simulink model "PLFrameGenerator"  (R2023a)
settings: Solver=FixedStepAuto  StartTime=0.0  StopTime=135e-7  RelTol=1e-3
model workspace (MAT data in the model file):
  G = [1  0  0  1  0  0  0  0  1  0  1  0  1  1  0  0  0  0  1  0  1  1  0  1  1  1  0  1  1  1  0  1; 0  1  0  1  0  1  0  1  0  1  0  1  0  1  0  1  0  1  0  1  0  1  0  1  0  1  0  1  0  1  0  1; 0  0  1  1  0  0  1  1  0  0  1  1  0  0  1  1  0  0  1  1  0  0  1  1  0  0  1  1  0  0  1  1; 0  0  0  0  1  1  1  1  0  0  0  0  1  1  1  1  0  0  0  0  1  1  1  1  0  0  0  0  1  1  1  1; 0  0  0  0  0  0  0  0  1  1  1  1  1  1  1  1  0  0  0  0  0  0  0  0  1  1  1  1  1  1  1  1; 0  0  0  0  0  0  0  0  0  0  0  0  0  0  0  0  1  1  1  1  1  1  1  1  1  1  1  1  1  1  1  1; 1  1  1  1  1  1  1  1  1  1  1  1  1  1  1  1  1  1  1  1  1  1  1  1  1  1  1  1  1  1  1  1]
  HDRShortDUMMY = Simulink.LookupTable
  HDRShortDUMMY.Table = Simulink.lookuptable.Table
  HDRShortDUMMY.Table.Value = [-0.707106781187-0.707106781187i -0.707106781187+0.707106781187i -0.707106781187-0.707106781187i 0.707106781187-0.707106781187i -0.707106781187-0.707106781187i 0.707106781187-0.707106781187i 0.707106781187+0.707106781187i -0.707106781187+0.707106781187i 0.707106781187+0.707106781187i -0.707106781187+0.707106781187i 0.707106781187+0.707106781187i 0.707106781187-0.707106781187i ... (64 elements, 64x1)]
  HDRShortDUMMY.Table.Dimensions = [64 1]
  HDRShortDUMMY.Table.DataType = 'auto'
  HDRShortDUMMY.Table.FieldName = 'Table'
  HDRShortDUMMY.Breakpoints = Simulink.lookuptable.Breakpoint
  HDRShortDUMMY.Breakpoints.TunableSizeName = 'N1'
  HDRShortDUMMY.Breakpoints.Dimensions = [0 0]
  HDRShortDUMMY.Breakpoints.DataType = 'auto'
  HDRShortDUMMY.Breakpoints.FieldName = 'BP1'
  HDRShortDUMMY.AllowMultipleInstancesOfTypeToHaveDifferentTableBreakpointSizes = 0
  HDRShortDUMMY.SupportTunableSize = 0
  HDRShortDUMMY.StructTypeInfo = Simulink.lookuptable.StructTypeInfo
  HDRShortDUMMY.StructTypeInfo.DataScope = 'Auto'
  PLSCLength = 90
  PilotMaxIdx = 1475
  PilotMinIdx = 1440
  Rsym = 10000000
  SNR = Simulink.Parameter
  SNR.Value = 50
  SNR.DataType = 'auto'
  SNR.Complexity = 'real'
  SNR.Dimensions = [1 1]
  SOFLength = 26
  debugHeaderGain = 2
  mwTaskManagerKernelLatency = 0
  up_coef = 2
undefined symbols (not defined in the file or in its folder): Add, magnitude, Shift
libraries: simulink x15, hdlsllib x14, dsphdlfiltering2 x4, embmathops x4, dspsigops x3, commrandsrc3 x1, commfilt2 x1, dsphdlmathfun2 x1, commchan3 x1
(part 1 of 2)
settings Model: SimulationMode=accelerator  ParameterArgumentNames=SNR  Creator=svdvl  LastModifiedBy=x
settings OptimizationCC: DefaultParameterBehavior=Inlined  EnhancedBackFolding=on  PassReuseOutputArgsAs=Individual arguments  ZeroExternalMemoryAtStartup=off  ZeroInternalMemoryAtStartup=off  MaxStackSize=64  OptimizeBlockOrder=speed  DifferentSizesBufferReuse=on  OptimizationCustomize=off  EfficientTunableParamExpr=on
settings DebuggingCC: SingleTaskRateTransMsg=error  ParameterTunabilityLossMsg=error
settings HardwareCC: ProdBitPerPointer=32  ProdBitPerSizeT=32  ProdBitPerPtrDiffT=32  ProdLargestAtomicFloat=None  ProdIntDivRoundTo=Undefined  ProdEndianess=Unspecified  ProdWordSize=32  ProdHWDeviceType=ASIC/FPGA->ASIC/FPGA  TargetBitPerPointer=64  TargetBitPerSizeT=64  TargetBitPerPtrDiffT=64  TargetLongLongMode=on  TargetIntDivRoundTo=Zero  TargetEndianess=LittleEndian  TargetWordSize=64  TargetHWDeviceType=Custom Processor->MATLAB Host Computer  ProdEqTarget=off  HardwareBoardFeatureSet=SoCBlockset
settings SFSimCC: MATLABDynamicMemAlloc=off
settings RTWCC: Description=Embedded Coder  SystemTargetFile=ert.tlc  HardwareBoard=Xilinx Kintex-7 KC705 development board  TemplateMakefile=ert_default_tmf
settings CodeAppCC: ForceParamTrailComments=on  IgnoreCustomStorageClasses=off  OperatorAnnotations=on  SimulinkDataObjDesc=on  SFDataObjDesc=on  InsertBlockDesc=on
settings ERTTargetCC: InlinedParameterPlacement=NonHierarchical

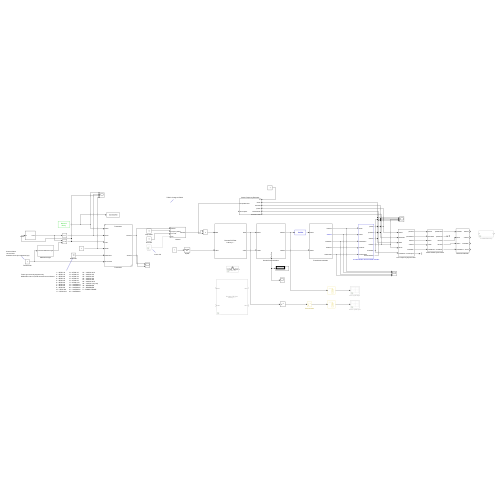
[thumbnail: Simulink's stored preview of the top-level diagram]
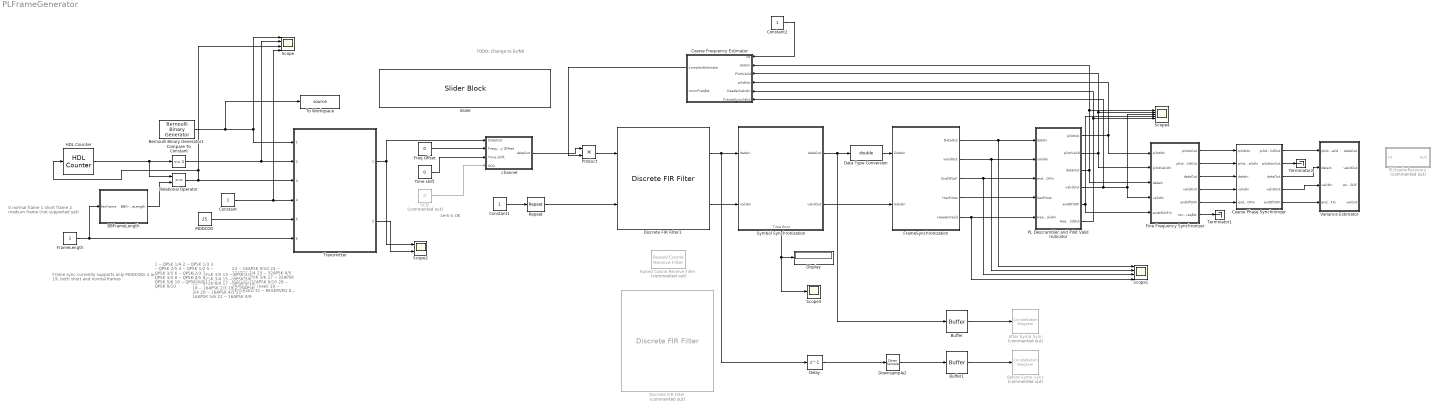
== system PLFrameGenerator ==
  note: Frame sync currently supports only
      | MODCODs 4 and 19, both short and normal frames
  note: 1e-6 is OK
  note: TODO: Change to Es/N0
  note: 23 -- 16APSK 9/10
      | 24 -- 32APSK 3/4
      | 25 -- 32APSK 4/5
      | 26 -- 32APSK 5/6
      | 27 -- 32APSK 8/9
      | 28 -- 32APSK 9/10
      | 29 -- 16APSK 1/2 (new)
      | 30 -- RESERVED
      | 31 -- RESERVED
      | 0 -- DUMMY FRAME
  note: 12 -- 8PSK 3/5
      | 13 -- 8PSK 2/3
      | 14 -- 8PSK 3/4
      | 15 -- 8PSK 5/6
      | 16 -- 8PSK 8/9
      | 17 -- 8PSK 9/10
      | 18 -- 16APSK 2/3
      | 19 -- 16APSK 3/4
      | 20 -- 16APSK 4/5
      | 21 -- 16APSK 5/6
      | 22 -- 16APSK 8/9
  note: 1 -- QPSK 1/4
      | 2 -- QPSK 1/3
      | 3 -- QPSK 2/5
      | 4 -- QPSK 1/2
      | 5 -- QPSK 3/5
      | 6 -- QPSK 2/3
      | 7 -- QPSK 3/4
      | 8 -- QPSK 4/5
      | 9 -- QPSK 5/6
      | 10 -- QPSK 8/9
      | 11 -- QPSK 9/10
  note: 0 normal frame
      | 1 short frame
      | 2 medium frame (not supported yet)
  After Symb Sync : ConstellationDiagram  Commented=on  WindowPosition=[1126.000000,74.000000,600.000000,600.000000,]  ScopeFrameLocation=window  DefaultConfigurationName=comm.scopes.ConstellationDiagramBlockCfg
  BBFrameLength : Subsystem
  Before Symb Sync : ConstellationDiagram  Commented=on  WindowPosition=[70.000000,95.000000,600.000000,600.000000,]  ScopeFrameLocation=window  DefaultConfigurationName=comm.scopes.ConstellationDiagramBlockCfg
  Bernoulli Binary Generator1 : commrandsrc3/Bernoulli Binary Generator  ProbabilityOfZero=0.5  SeedSource=Auto  Seed=0  SampleTime=1/Rsym/8  SamplesPerFrame=1  OutputDataType=boolean  SimulateUsing=Code generation
  Buffer : Buffer  N=1000  OutputFrames=off
  Buffer1 : Buffer  N=1000  OutputFrames=off
  Coarse Frequency Estimator : Subsystem
  Coarse Phase Synchronizer : Subsystem
  Compare To Constant : simulink/Logic and Bit Operations/Compare To Constant  relop===  const=1  OutDataTypeStr=boolean
  Constant : Constant  OutDataTypeStr=boolean  SampleTime=1/Rsym/8
  Constant1 : Constant  OutDataTypeStr=boolean  SampleTime=-1
  Constant2 : Constant  SampleTime=-1
  Data Type Conversion : DataTypeConversion  OutDataTypeStr=double  SaturateOnIntegerOverflow=off  RndMeth=Floor
  Delay : Delay  DelayLength=1
  Discrete FIR Filter : dsphdlfiltering2/Discrete FIR Filter  Commented=on  NumeratorSource=Property  Numerator="[-0.00285820997079789\t0.00137733032508190\t0.00315455482520775\t-0.00356415296709377\t-0.00206211933009069\t0.00514477794743620\t-0.000825518525453186\t-0.00481272795526686\t0.00560922270003514\t0.000910808542107733\t-0.0120044818773511\t0.00862996822246556\t0.0193455321229390\t-0.0268242332250627\t-0.0266806119948057\t0.0600224093867556\t0.0329422984385442\t-0.130628932045810\t-0.0371565869289195\t0.443442194227448\t0.745765109300838\t0.443442194227448\t-0.0371565869289195\t-0.130628932045810\t0.0329422984385442\t0.0600224093867556\t-0.0266806119948057\t-0.0268242332250627\t0.0193455321229390\t0.00862996822246556\t-0.0120044818773511\t0.000910808542107733\t0.00560922270003514\t-0.00481272795526686\t-0.000825518525453186\t0.00514477794743620\t-0.00206211933009069\t-0.00356415296709377\t0.00315455482520775\t0.00137733032508190\t-0.00285820997079789]"  NumeratorPrototype=[]  FilterStructure=Direct form systolic  SerializationOption=Minimum number of cycles between valid input samples  NumCycles=2  NumberOfMultipliers=2  SimulateUsing=Code generation  roundingMode=Floor  overflowMode=off  CoefficientsDataTypeStr=Inherit: Same word length as input  OutputDataTypeStr=Inherit: Same word length as input  ResetInputPort=off  HDLGlobalReset=off
  Discrete FIR Filter1 : dsphdlfiltering2/Discrete FIR Filter  NumeratorSource=Property  Numerator="[-0.00285820997079789\t0.00137733032508190\t0.00315455482520775\t-0.00356415296709377\t-0.00206211933009069\t0.00514477794743620\t-0.000825518525453186\t-0.00481272795526686\t0.00560922270003514\t0.000910808542107733\t-0.0120044818773511\t0.00862996822246556\t0.0193455321229390\t-0.0268242332250627\t-0.0266806119948057\t0.0600224093867556\t0.0329422984385442\t-0.130628932045810\t-0.0371565869289195\t0.443442194227448\t0.745765109300838\t0.443442194227448\t-0.0371565869289195\t-0.130628932045810\t0.0329422984385442\t0.0600224093867556\t-0.0266806119948057\t-0.0268242332250627\t0.0193455321229390\t0.00862996822246556\t-0.0120044818773511\t0.000910808542107733\t0.00560922270003514\t-0.00481272795526686\t-0.000825518525453186\t0.00514477794743620\t-0.00206211933009069\t-0.00356415296709377\t0.00315455482520775\t0.00137733032508190\t-0.00285820997079789]"  NumeratorPrototype=[]  FilterStructure=Direct form systolic  SerializationOption=Minimum number of cycles between valid input samples  NumCycles=2  NumberOfMultipliers=2  SimulateUsing=Code generation  roundingMode=Floor  overflowMode=off  CoefficientsDataTypeStr=Inherit: Same word length as input  OutputDataTypeStr=Inherit: Same word length as input  ResetInputPort=off  HDLGlobalReset=off
  Display : Display
  Downsample2 : DownSample  RateOptions=Allow multirate processing
  Fine Frequency Synchronizer : Subsystem
  FrameLength : Constant  OutDataTypeStr=fixdt(0,2,0)  SampleTime=1/Rsym/8
  FrameSynchronization : Subsystem
  Freq Offset : Constant  Value=0
  HDL Counter : hdlsllib/Sources/HDL Counter  CountType=Count limited  CountInit=1  CountStep=1  CountMax=64800  CountFromType=Initial value  CountFrom=1  CountResetPort=on  CountLoadPort=off  CountEnbPort=off  CountDirPort=off  CountHitOutputPort=off  CountDataType=Unsigned  CountWordLen=16  CountFracLen=0  CountSampTime=1/Rsym/8
  MODCOD : Constant  Value=25  VectorParams1D=off  OutDataTypeStr=fixdt(0, 5, 0)  SampleTime=1/Rsym/8
  PL Descrambler and Pilot Valid Indicator : Subsystem
  PLHeaderRecovery : Subsystem  Commented=on
  Product : Product
  Raised Cosine Receive Filter : commfilt2/Raised Cosine Receive Filter  Commented=on  filtType=Square root  R=0.2  filtSpan=20  N=2  downFactor=1  downOffset=0  filterGain=1  InputProcessing=Columns as channels (frame based)  RateOptions=Enforce single-rate processing  framing=Mute  checkCoeff=on  variableName=rcRxFilt  currentFiltSpan=10  D=5  inputOffset=0  sampMode=Mute  saveAsFlag=0  rateMode=Downsampling  checkGain=Normalized  launchFVT=on  roundingMode=Floor  overflowMode=off  coeffDataTypeStr=Inherit: Same word length as input  coeffMin=[]  coeffMax=[]  coeffLastDataTypeStr=Inherit: Same word length as input  accumDataTypeStr=Inherit: Same as product output  accumLastDataTypeStr=Inherit: Same as product output  outputDataTypeStr=Inherit: Same as accumulator  outputMin=[]  outputMax=[]  outputLastDataTypeStr=Inherit: Same as accumulator
  Relational Operator : RelationalOperator  Operator===  OutDataTypeStr=boolean  RndMeth=Simplest  InputSameDT=off
  Repeat : dspsigops/Repeat  FactorSource=Dialog parameter  N=2  Nmax=16  RateOptions=Allow multirate processing  ic=0  mode=Unused parameter value
      settings: LibrarySourceBlock=dsphdlsupportsigops/Repeat
  SCO : Constant  Commented=on  Value=0  SampleTime=1/2/Rsym
  Scope : Scope  NumInputPorts=4
  Scope1 : Scope  NumInputPorts=4
  Scope2 : Scope  NumInputPorts=2
  Scope3 : Scope
  Scope4 : Scope  NumInputPorts=5
  Slider : SliderBlock  ScaleMin=-10  ScaleMax=50
  Symbol Synchronization : Subsystem
      settings: PortSchema="{\"entries\":[{\"content\":{\"sides\":[{\"content\":{\"connectorIds\":[\"In1\",\"In2\"]},\"type\":\"ConnectorPlacement.EquallySpacedRectSide\",\"uuid\":\"e58971f0-ac8c-4c81-a411-2548e0157a31\"},{\"content\":{\"connectorIds\":[\"Out1\",\"Out2\"],\"side\":\"RIGHT\"},\"type\":\"ConnectorPlacement.EquallySpacedRectSide\",\"uuid\":\"61e7e244-d935-4f43-ae64-0dd24601d7d6\"},{\"content\":{\"connectorIds\":[],\"side\":\"TOP\"},\"type\":\"ConnectorPlacement.EquallySpacedRectSide\",\"uuid\":\"96280ba8-4d2f-4f61-8153-d5e9f705abd5\"},{\"content\":{\"connectorIds\":[\"Out3\"],\"side\":\"BOTTOM\"},\"type\":\"ConnectorPlacement.EquallySpacedRectSide\",\"uuid\":\"1f39d276-a9ad-4a31-a5cc-29fbe76e4b28\"}]},\"type\":\"ConnectorPlacement.EquallySpacedConnector\",\"uuid\":\"475f41bb-1527-498a-b7fd-c47195976015\"}],\"packageUris\":[\"http://schema.mathworks.com/mf0/Connector/R2020b\"],\"version\":\"1.0\"}"
  Terminator1 : Terminator
  Terminator2 : Terminator
  Time shift : Constant  Value=0  SampleTime=-1
  To Workspace : ToWorkspace  VariableName=source  SampleTime=-1
  Transmitter : Subsystem  ReferencedSubsystem=Transmitter
  Variance Estimator : Subsystem
  channel : Subsystem
  wires:
  Bernoulli Binary Generator1/1 -> To Workspace/1, Transmitter/1, Scope/1
  Constant/1 -> Transmitter/4, Scope/4
  FrameLength/1 -> Transmitter/6, BBFrameLength/1(fecframe)
  Compare To Constant/1 -> Transmitter/2, Scope/2
  HDL Counter/1 -> Compare To Constant/1, Relational Operator/1
  BBFrameLength/1(BBFrameLength) -> Relational Operator/2
  MODCOD/1 -> Transmitter/5
  Relational Operator/1 -> Transmitter/3, Scope/3, HDL Counter/1
  Transmitter/1 -> Scope2/1, channel/1(DataOut)
  Transmitter/2 -> Scope2/2
  Constant1/1 -> Repeat/1
  Buffer/1 -> After Symb Sync/1
  Symbol Synchronization/1(dataOut) -> Data Type Conversion/1, Buffer/1
  FrameSynchronization/1(DataOut) -> Scope1/1, PL Descrambler and Pilot Valid Indicator/1(dataIn)
  FrameSynchronization/2(ValidOut) -> Scope1/2, PL Descrambler and Pilot Valid Indicator/2(validIn)
  FrameSynchronization/3(EndOfSoF) -> Scope1/3, PL Descrambler and Pilot Valid Indicator/3(endOfSOFIn)
  Data Type Conversion/1 -> FrameSynchronization/1(DataIn)
  Symbol Synchronization/2(validOut) -> FrameSynchronization/2(ValidIn)
  Freq Offset/1 -> channel/2(Frequency Offset)
  Time shift/1 -> channel/3(Time shift)
  SCO/1 -> channel/4(SCO)
  Buffer1/1 -> Before Symb Sync/1
  Downsample2/1 -> Buffer1/1
  Product/1 -> Discrete FIR Filter1/1
  Discrete FIR Filter1/1 -> Delay/1, Symbol Synchronization/1(dataIn)
  Discrete FIR Filter1/2 -> Symbol Synchronization/2(validIn)
  Repeat/1 -> Discrete FIR Filter1/2
  Delay/1 -> Downsample2/1
  Symbol Synchronization/3(Time Error) -> Scope3/1, Display/1
  FrameSynchronization/4(HasPilots) -> PL Descrambler and Pilot Valid Indicator/4(hasPilots)
  PL Descrambler and Pilot Valid Indicator/1(pilotIdx) -> Fine Frequency Synchronizer/1(pilotIdx), Coarse Frequency Estimator/4(pilotIdx)
  PL Descrambler and Pilot Valid Indicator/2(pilotValid) -> Fine Frequency Synchronizer/2(pilotValidIn), Coarse Frequency Estimator/3(PilotValid), Scope4/2
  PL Descrambler and Pilot Valid Indicator/3(dataOut) -> Coarse Frequency Estimator/2(dataIn), Scope4/1, Fine Frequency Synchronizer/3(dataIn)
  Constant2/1 -> Coarse Frequency Estimator/1(rst)
  Coarse Frequency Estimator/1(complexEstimate) -> Product/2
  PL Descrambler and Pilot Valid Indicator/4(validOut) -> Fine Frequency Synchronizer/4(validIn), Scope4/3, Coarse Frequency Estimator/6(FrameSyncValid)
  PL Descrambler and Pilot Valid Indicator/5(endOfSOF) -> Scope4/4, Fine Frequency Synchronizer/5(endofSOFIn)
  Fine Frequency Synchronizer/1(pilotsOut) -> Coarse Phase Synchronizer/1(pilotIdx)
  Fine Frequency Synchronizer/2(pilotValidOut) -> Coarse Phase Synchronizer/2(pilotValidIn)
  Fine Frequency Synchronizer/3(dataOut) -> Coarse Phase Synchronizer/3(dataIn)
  Fine Frequency Synchronizer/4(validOut) -> Coarse Phase Synchronizer/4(validIn)
  Fine Frequency Synchronizer/5(endOfSOF) -> Coarse Phase Synchronizer/5(endOfSOFIn)
  Fine Frequency Synchronizer/6(normFreqEst) -> Terminator1/1
  Coarse Phase Synchronizer/1(pilotValidOut) -> Variance Estimator/1(pilotValid)
  Coarse Phase Synchronizer/3(dataOut) -> Variance Estimator/2(dataIn)
  Coarse Phase Synchronizer/4(validOut) -> Variance Estimator/3(validIn)
  Coarse Phase Synchronizer/5(endOfSOF) -> Variance Estimator/4(endOfSOFIn)
  Coarse Phase Synchronizer/2(pilotIdxOut) -> Terminator2/1
  channel/1(dataOut) -> Product/1
  FrameSynchronization/5(HeaderValid) -> PL Descrambler and Pilot Valid Indicator/5(HeaderValidIn), Scope1/4
  PL Descrambler and Pilot Valid Indicator/6(HeaderValidOut) -> Coarse Frequency Estimator/5(HeaderValidIn), Scope4/5

== system PLFrameGenerator/BBFrameLength ==
  note: Number of bits in a frame
  note: 0 normal frame
      | 1 short frame
      | 2 medium frame
  fecframe : Inport
  Display : Display
  Medium Frame bit length : Constant  Value=32400
  Multiport Switch : MultiPortSwitch  DataPortOrder=Zero-based contiguous  zeroidx=on  SaturateOnIntegerOverflow=off  InputSameDT=off
  Normal Frame bit length : Constant  Value=64800
  Short Frame bit length : Constant  Value=16200
  BBFrameLength : Outport
  wires:
  fecframe/1 -> Multiport Switch/1
  Multiport Switch/1 -> Display/1, BBFrameLength/1
  Medium Frame bit length/1 -> Multiport Switch/4
  Short Frame bit length/1 -> Multiport Switch/3
  Normal Frame bit length/1 -> Multiport Switch/2

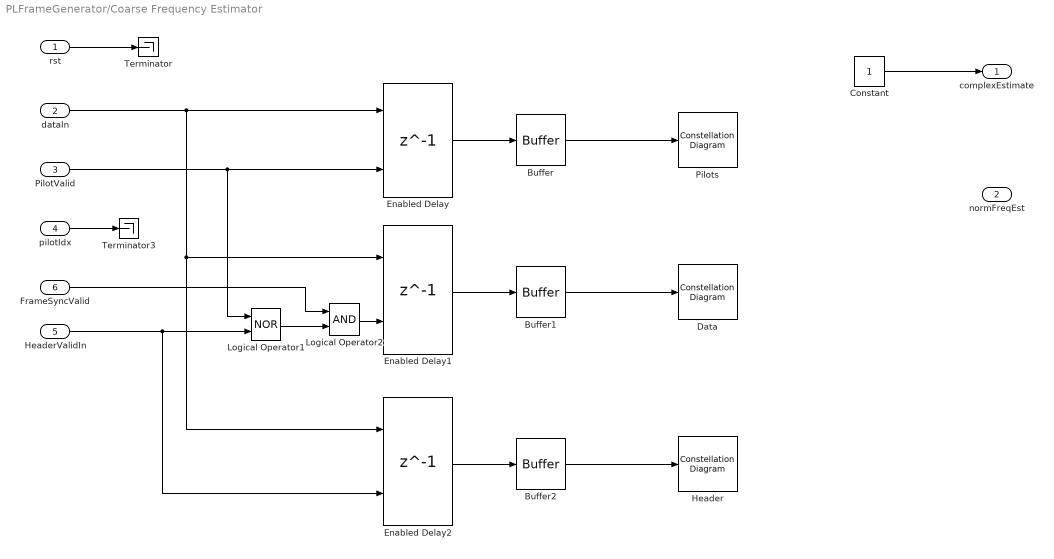
== system PLFrameGenerator/Coarse Frequency Estimator ==
  rst : Inport
  dataIn : Inport  Port=2
  PilotValid : Inport  Port=3
  pilotIdx : Inport  Port=4
  HeaderValidIn : Inport  Port=5
  FrameSyncValid : Inport  Port=6
  Buffer : Buffer  N=4000  OutputFrames=off
  Buffer1 : Buffer  N=4000  OutputFrames=off
  Buffer2 : Buffer  N=4000  OutputFrames=off
  Constant : Constant  SampleTime=1/Rsym/2
  Data : ConstellationDiagram  WindowPosition=[1243.000000,145.000000,600.000000,600.000000,]  ScopeFrameLocation=window  DefaultConfigurationName=comm.scopes.ConstellationDiagramBlockCfg
  Enabled Delay : Delay  DelayLength=1  ShowEnablePort=on
      settings: InputPortMap=u0,e6
  Enabled Delay1 : Delay  DelayLength=1  ShowEnablePort=on
      settings: InputPortMap=u0,e6
  Enabled Delay2 : Delay  DelayLength=1  ShowEnablePort=on
      settings: InputPortMap=u0,e6
  Header : ConstellationDiagram  WindowPosition=[629.000000,144.000000,600.000000,600.000000,]  ScopeFrameLocation=window  DefaultConfigurationName=comm.scopes.ConstellationDiagramBlockCfg
  Logical Operator1 : Logic  Operator=NOR  AllPortsSameDT=off  OutDataTypeStr=boolean
  Logical Operator2 : Logic  AllPortsSameDT=off  OutDataTypeStr=boolean
  Pilots : ConstellationDiagram  WindowPosition=[9.000000,145.000000,600.000000,600.000000,]  ScopeFrameLocation=window  DefaultConfigurationName=comm.scopes.ConstellationDiagramBlockCfg
  Terminator : Terminator
  Terminator3 : Terminator
  complexEstimate : Outport
  normFreqEst : Outport  Port=2
  wires:
  Constant/1 -> complexEstimate/1
  rst/1 -> Terminator/1
  dataIn/1 -> Enabled Delay2/1, Enabled Delay1/1, Enabled Delay/1
  pilotIdx/1 -> Terminator3/1
  Enabled Delay/1 -> Buffer/1
  Enabled Delay1/1 -> Buffer1/1
  Buffer/1 -> Pilots/1
  Buffer1/1 -> Data/1
  PilotValid/1 -> Enabled Delay/2, Logical Operator1/1
  HeaderValidIn/1 -> Enabled Delay2/2, Logical Operator1/2
  Enabled Delay2/1 -> Buffer2/1
  Buffer2/1 -> Header/1
  Logical Operator2/1 -> Enabled Delay1/2
  Logical Operator1/1 -> Logical Operator2/2
  FrameSyncValid/1 -> Logical Operator2/1

== system PLFrameGenerator/Coarse Phase Synchronizer ==
  pilotIdx : Inport
  pilotValidIn : Inport  Port=2
  dataIn : Inport  Port=3
  validIn : Inport  Port=4
  endOfSOFIn : Inport  Port=5
  pilotValidOut : Outport
  pilotIdxOut : Outport  Port=2
  dataOut : Outport  Port=3
  validOut : Outport  Port=4
  endOfSOF : Outport  Port=5
  wires:
  pilotIdx/1 -> pilotValidOut/1
  pilotValidIn/1 -> pilotIdxOut/1
  dataIn/1 -> dataOut/1
  validIn/1 -> validOut/1
  endOfSOFIn/1 -> endOfSOF/1

== system PLFrameGenerator/Fine Frequency Synchronizer ==
  pilotIdx : Inport
  pilotValidIn : Inport  Port=2
  dataIn : Inport  Port=3
  validIn : Inport  Port=4
  endofSOFIn : Inport  Port=5
  Constant : Constant  Value=0  SampleTime=-1
  pilotsOut : Outport
  pilotValidOut : Outport  Port=2
  dataOut : Outport  Port=3
  validOut : Outport  Port=4
  endOfSOF : Outport  Port=5
  normFreqEst : Outport  Port=6
  wires:
  pilotIdx/1 -> pilotsOut/1
  pilotValidIn/1 -> pilotValidOut/1
  dataIn/1 -> dataOut/1
  validIn/1 -> validOut/1
  endofSOFIn/1 -> endOfSOF/1
  Constant/1 -> normFreqEst/1

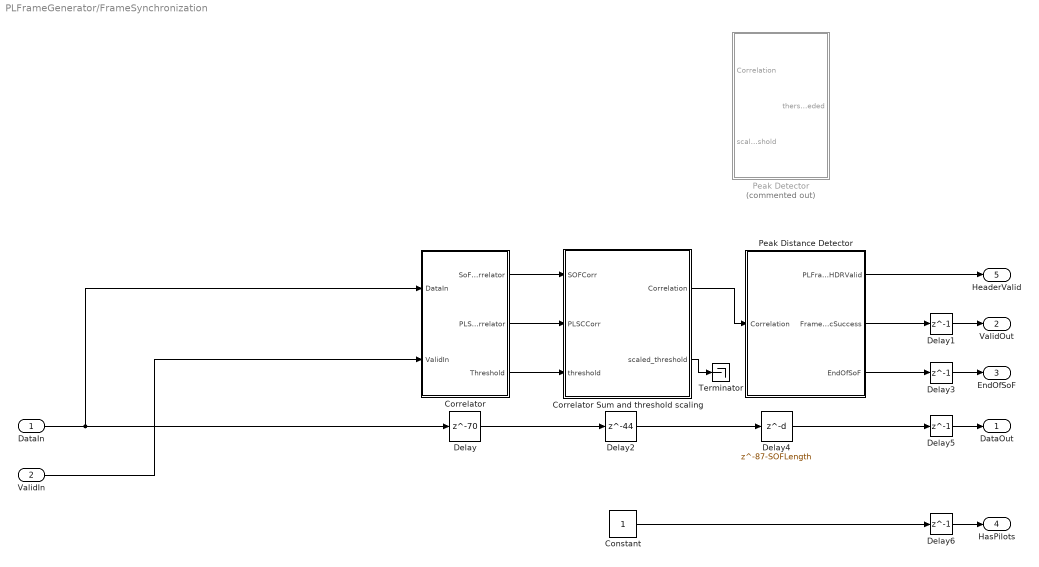
== system PLFrameGenerator/FrameSynchronization ==
  DataIn : Inport
  ValidIn : Inport  Port=2
  Constant : Constant  OutDataTypeStr=boolean  SampleTime=1/Rsym
  Correlator : Subsystem
  Correlator Sum and threshold scaling : Subsystem
  Delay : Delay  DelayLength=70  SampleTime=1/Rsym
  Delay{1,3,5..6} (4 alike) : Delay  DelayLength=1
  Delay2 : Delay  DelayLength=44  SampleTime=1/Rsym
  Delay4 : Delay  DelayLength=87-SOFLength  SampleTime=1/Rsym
  Peak Detector : Subsystem  Commented=on
  Peak Distance Detector : Subsystem
      settings: PortSchema="{\"entries\":[{\"content\":{\"sides\":[{\"content\":{\"connectorIds\":[]},\"type\":\"ConnectorPlacement.EquallySpacedRectSide\",\"uuid\":\"dfc8d0c6-fd53-4519-953d-8693d3949103\"},{\"content\":{\"connectorIds\":[],\"side\":\"RIGHT\"},\"type\":\"ConnectorPlacement.EquallySpacedRectSide\",\"uuid\":\"3ac206ed-ff95-43ab-a46f-2cfd8d306125\"},{\"content\":{\"connectorIds\":[\"In1\"],\"side\":\"TOP\"},\"type\":\"ConnectorPlacement.EquallySpacedRectSide\",\"uuid\":\"3940d45e-d68d-40b5-a0eb-a815ef26171f\"},{\"content\":{\"connectorIds\":[\"Out1\",\"Out2\",\"Out3\"],\"side\":\"BOTTOM\"},\"type\":\"ConnectorPlacement.EquallySpacedRectSide\",\"uuid\":\"2f4bb652-8288-4055-bc48-5789bd3d5e4d\"}]},\"type\":\"ConnectorPlacement.EquallySpacedConnector\",\"uuid\":\"2a412ce9-0bfc-474d-ac66-4698babe86c7\"}],\"packageUris\":[\"http://schema.mathworks.com/mf0/Connector/R2020b\"],\"version\":\"1.0\"}"
  Terminator : Terminator
  DataOut : Outport
  ValidOut : Outport  Port=2
  EndOfSoF : Outport  Port=3
  HasPilots : Outport  Port=4
  HeaderValid : Outport  Port=5
  wires:
  DataIn/1 -> Correlator/1(DataIn), Delay/1
  ValidIn/1 -> Correlator/2(ValidIn)
  Correlator/1(SoFCorrelator) -> Correlator Sum and threshold scaling/1(SOFCorr)
  Correlator/2(PLSCCorrelator) -> Correlator Sum and threshold scaling/2(PLSCCorr)
  Correlator/3(Threshold) -> Correlator Sum and threshold scaling/3(threshold)
  Delay/1 -> Delay2/1
  Delay2/1 -> Delay4/1
  Constant/1 -> Delay6/1
  Peak Distance Detector/1(EndOfSoF) -> Delay3/1
  Correlator Sum and threshold scaling/2(scaled_threshold) -> Terminator/1
  Correlator Sum and threshold scaling/1(Correlation) -> Peak Distance Detector/1(Correlation)
  Delay4/1 -> Delay5/1
  Peak Distance Detector/2(FrameSyncSuccess) -> Delay1/1
  Peak Distance Detector/3(PLFrameHDRValid) -> HeaderValid/1
  Delay3/1 -> EndOfSoF/1
  Delay1/1 -> ValidOut/1
  Delay5/1 -> DataOut/1
  Delay6/1 -> HasPilots/1

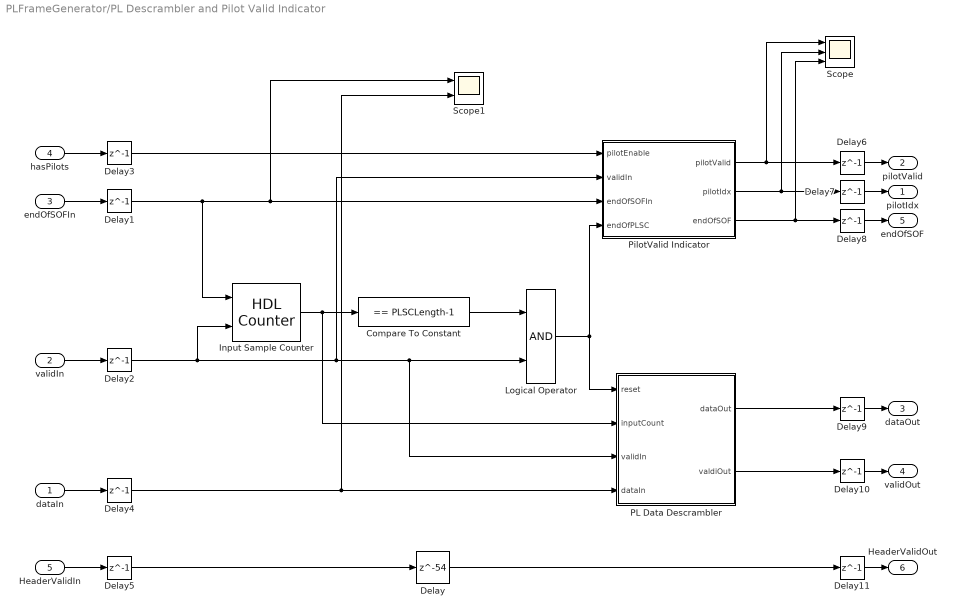
== system PLFrameGenerator/PL Descrambler and Pilot Valid Indicator ==
  dataIn : Inport
  validIn : Inport  Port=2
  endOfSOFIn : Inport  Port=3
  hasPilots : Inport  Port=4
  HeaderValidIn : Inport  Port=5
  Compare To Constant : simulink/Logic and Bit Operations/Compare To Constant  relop===  const=PLSCLength-1  OutDataTypeStr=boolean
  Delay : Delay  DelayLength=54
  Delay{1..11} (11 alike) : Delay  DelayLength=1
  Input Sample Counter : hdlsllib/Sources/HDL Counter  CountType=Free running  CountInit=0  CountStep=1  CountMax=25  CountFromType=Initial value  CountFrom=0  CountResetPort=on  CountLoadPort=off  CountEnbPort=on  CountDirPort=off  CountHitOutputPort=off  CountDataType=Unsigned  CountWordLen=32  CountFracLen=0  CountSampTime=1
  Logical Operator : Logic  AllPortsSameDT=off  OutDataTypeStr=boolean
  PL Data Descrambler : Subsystem
  PilotValid Indicator : Subsystem
  Scope : Scope  NumInputPorts=3
  Scope1 : Scope  NumInputPorts=2
  pilotIdx : Outport
  pilotValid : Outport  Port=2
  dataOut : Outport  Port=3
  validOut : Outport  Port=4
  endOfSOF : Outport  Port=5
  HeaderValidOut : Outport  Port=6
  wires:
  endOfSOFIn/1 -> Delay1/1
  validIn/1 -> Delay2/1
  Input Sample Counter/1 -> PL Data Descrambler/2(inputCount), Compare To Constant/1
  Compare To Constant/1 -> Logical Operator/1
  Logical Operator/1 -> PilotValid Indicator/4(endOfPLSC), PL Data Descrambler/1(reset)
  dataIn/1 -> Delay4/1
  PL Data Descrambler/1(dataOut) -> Delay9/1
  PL Data Descrambler/2(valdiOut) -> Delay10/1
  hasPilots/1 -> Delay3/1
  PilotValid Indicator/1(pilotValid) -> Scope/1, Delay6/1
  PilotValid Indicator/2(pilotIdx) -> Scope/2, Delay7/1
  PilotValid Indicator/3(endOfSOF) -> Scope/3, Delay8/1
  Delay3/1 -> PilotValid Indicator/1(pilotEnable)
  Delay1/1 -> Input Sample Counter/1, Scope1/1, PilotValid Indicator/3(endOfSOFIn)
  Delay2/1 -> PilotValid Indicator/2(validIn), PL Data Descrambler/3(validIn), Logical Operator/2, Input Sample Counter/2
  Delay4/1 -> Scope1/2, PL Data Descrambler/4(dataIn)
  HeaderValidIn/1 -> Delay5/1
  Delay/1 -> Delay11/1
  Delay5/1 -> Delay/1
  Delay6/1 -> pilotValid/1
  Delay7/1 -> pilotIdx/1
  Delay8/1 -> endOfSOF/1
  Delay9/1 -> dataOut/1
  Delay10/1 -> validOut/1
  Delay11/1 -> HeaderValidOut/1

== system PLFrameGenerator/PLHeaderRecovery ==
  In1 : Inport
  Out1 : Outport
  wires:
  In1/1 -> Out1/1

== system PLFrameGenerator/Symbol Synchronization ==
  dataIn : Inport  PortDimensions=1
  validIn : Inport  Port=2
  Constant : Constant  Commented=on  Value=-1  SampleTime=-1
  Cubic Interpolator : Subsystem
      settings: PortSchema="{\"entries\":[{\"content\":{\"sides\":[{\"content\":{\"connectorIds\":[\"In1\"]},\"type\":\"ConnectorPlacement.EquallySpacedRectSide\",\"uuid\":\"e185856d-5f81-4c71-aeba-8657e8be69b7\"},{\"content\":{\"connectorIds\":[\"Out1\"],\"side\":\"RIGHT\"},\"type\":\"ConnectorPlacement.EquallySpacedRectSide\",\"uuid\":\"487ec109-4505-4025-a071-939a946bead6\"},{\"content\":{\"connectorIds\":[\"In2\"],\"side\":\"TOP\"},\"type\":\"ConnectorPlacement.EquallySpacedRectSide\",\"uuid\":\"bdbbf84f-c060-4097-b440-093ef9dcf44f\"},{\"content\":{\"connectorIds\":[],\"side\":\"BOTTOM\"},\"type\":\"ConnectorPlacement.EquallySpacedRectSide\",\"uuid\":\"14959837-ab14-4ae0-ae0e-9624de46668b\"}]},\"type\":\"ConnectorPlacement.EquallySpacedConnector\",\"uuid\":\"80c256de-e921-4425-90d6-76c464211f17\"}],\"packageUris\":[\"http://schema.mathworks.com/mf0/Connector/R2020b\"],\"version\":\"1.0\"}"
  Downsample1 : DownSample  RateOptions=Allow multirate processing
  Downsample2 : DownSample  RateOptions=Allow multirate processing
  Linear Interpolator : Subsystem  Commented=on
      settings: PortSchema="{\"entries\":[{\"content\":{\"sides\":[{\"content\":{\"connectorIds\":[\"In1\"]},\"type\":\"ConnectorPlacement.EquallySpacedRectSide\",\"uuid\":\"e185856d-5f81-4c71-aeba-8657e8be69b7\"},{\"content\":{\"connectorIds\":[\"Out1\"],\"side\":\"RIGHT\"},\"type\":\"ConnectorPlacement.EquallySpacedRectSide\",\"uuid\":\"487ec109-4505-4025-a071-939a946bead6\"},{\"content\":{\"connectorIds\":[\"In2\"],\"side\":\"TOP\"},\"type\":\"ConnectorPlacement.EquallySpacedRectSide\",\"uuid\":\"bdbbf84f-c060-4097-b440-093ef9dcf44f\"},{\"content\":{\"connectorIds\":[],\"side\":\"BOTTOM\"},\"type\":\"ConnectorPlacement.EquallySpacedRectSide\",\"uuid\":\"14959837-ab14-4ae0-ae0e-9624de46668b\"}]},\"type\":\"ConnectorPlacement.EquallySpacedConnector\",\"uuid\":\"80c256de-e921-4425-90d6-76c464211f17\"}],\"packageUris\":[\"http://schema.mathworks.com/mf0/Connector/R2020b\"],\"version\":\"1.0\"}"
  TED : Subsystem
  unwrapper : Subsystem
  dataOut : Outport
  validOut : Outport  Port=2
  Time Error : Outport  Port=3
  wires:
  dataIn/1 -> Cubic Interpolator/1(x), TED/1(dataIn)
  validIn/1 -> Downsample2/1
  TED/1(mu) -> unwrapper/1(In1)
  Cubic Interpolator/1(dataOut) -> Downsample1/1
  unwrapper/1(Output) -> Cubic Interpolator/2(mu), Time Error/1
  Downsample1/1 -> dataOut/1
  Downsample2/1 -> validOut/1

== system PLFrameGenerator/Variance Estimator ==
  pilotValid : Inport
  dataIn : Inport  Port=2
  validIn : Inport  Port=3
  endOfSOFIn : Inport  Port=4
  Constant : Constant  Value=0  SampleTime=-1
  Terminator : Terminator
  dataOut : Outport
  validOut : Outport  Port=2
  endOfSOF : Outport  Port=3
  varOut : Outport  Port=4
  wires:
  dataIn/1 -> dataOut/1
  validIn/1 -> validOut/1
  endOfSOFIn/1 -> endOfSOF/1
  pilotValid/1 -> Terminator/1
  Constant/1 -> varOut/1

== system PLFrameGenerator/channel ==
  DataOut : Inport
  Frequency Offset : Inport  Port=2
  Time shift : Inport  Port=3
  SCO : Inport  Port=4
  AWGN Channel : commchan3/AWGN Channel  LegacyMode=on  NoiseMethod="Signal to noise ratio  (SNR)"  noiseMode="Signal to noise ratio  (SNR)"  EbNo=15  EsNo=10  SNR=1.15516062884484  BitsPerSymbol=1  SignalPower=1  SamplesPerSymbol=1  SymbolPeriod=1  VarianceSource=Parameter  Variance=1  RandomStream=Global stream  Seed=67  SimulateUsing=Code generation
  Add : Sum
  Add Constant : Bias  Bias=199  SaturateOnIntegerOverflow=off
  Data Type Conversion : DataTypeConversion  OutDataTypeStr=double  SaturateOnIntegerOverflow=off  RndMeth=Floor
  Data Type Conversion1 : DataTypeConversion  Commented=through  OutDataTypeStr=fixdt(1, 18, 14)  SaturateOnIntegerOverflow=off  RndMeth=Floor
  Sum : Sum  Inputs=|++
  Unit Delay : UnitDelay  SampleTime=-1  HasFrameUpgradeWarning=on
  Variable Fractional Delay : dspsigops/Variable Fractional Delay  mode=OBSOLETE  modeActive=FIR  L=200  FarrowL=4  R=110  alpha=1  dmax=220  ic=0  noDFT=off  fallbackFIR=Clip to the minimum value necessary for centered kernel  fallbackFarrow=Clip to the minimum value necessary for centered kernel  roundingMode=Zero  overflowMode=off
  dataOut : Outport
  wires:
  DataOut/1 -> Data Type Conversion/1
  AWGN Channel/1 -> Data Type Conversion1/1
  Data Type Conversion1/1 -> dataOut/1
  Variable Fractional Delay/1 -> AWGN Channel/1
  Data Type Conversion/1 -> Variable Fractional Delay/1
  Time shift/1 -> Add Constant/1
  Add Constant/1 -> Sum/1
  Sum/1 -> Variable Fractional Delay/2
  SCO/1 -> Add/1
  Add/1 -> Unit Delay/1, Sum/2
  Unit Delay/1 -> Add/2

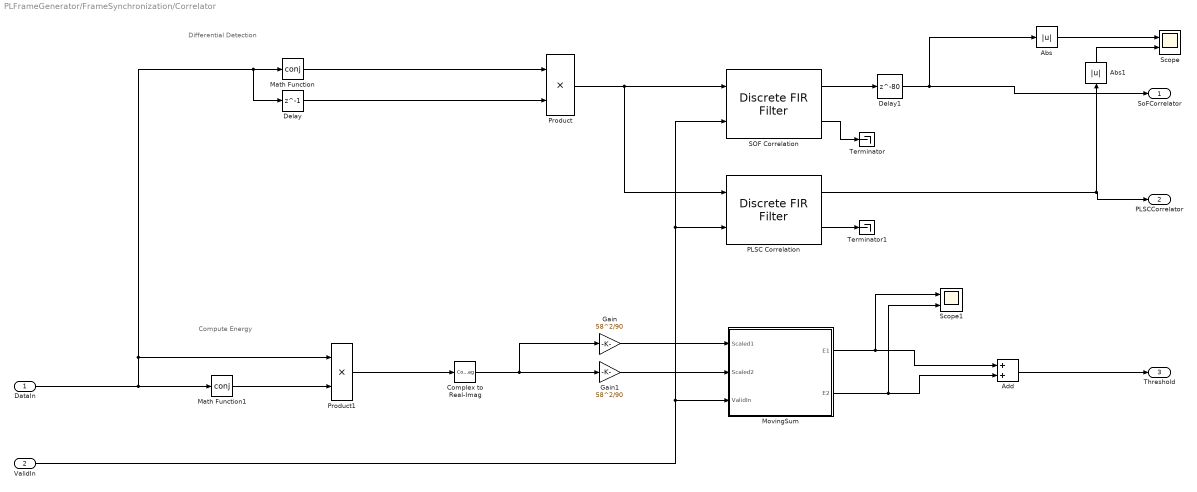
== system PLFrameGenerator/FrameSynchronization/Correlator ==
  note: Differential Detection
  note: Compute Energy
  DataIn : Inport
  ValidIn : Inport  Port=2
  Abs : Abs  SaturateOnIntegerOverflow=off
  Abs1 : Abs  SaturateOnIntegerOverflow=off
  Add : Sum
  Complex to Real-Imag : ComplexToRealImag  Output=Real
  Delay : Delay  DelayLength=1
  Delay1 : Delay  DelayLength=80
  Gain : Gain  Gain=58^2/90  OutDataTypeStr=double
  Gain1 : Gain  Gain=58^2/90  OutDataTypeStr=double
  Math Function : Math  Operator=conj
  Math Function1 : Math  Operator=conj
  MovingSum : Subsystem
  PLSC Correlation : dsphdlfiltering2/Discrete FIR Filter  NumeratorSource=Property  Numerator="flip([0.00207587049212865 + 1.00237167975181i\t0.00000000000000 + 0.00000000000000i\t8.97841895338702e-05 + 1.00037166900777i\t0.00000000000000 + 0.00000000000000i\t-0.00150009862867717 - 1.00261172640641i\t0.00000000000000 + 0.00000000000000i\t-0.00186313527990301 + 0.996924303079438i\t0.00000000000000 + 0.00000000000000i\t-0.00176874510379926 - 0.998123746787447i\t0.00000000000000 + 0.00000000000000i\t0.00351825220295110 + 1.00243783464914i\t0.00000000000000 + 0.00000000000000i\t-0.00104923899487630 - 1.00212768647515i\t0.00000000000000 + 0.00000000000000i\t-9.08941366732918e-05 - 1.00279065976558i\t0.00000000000000 + 0.00000000000000i\t0.000264511267563772 + 0.994765012470802i\t0.00000000000000 + 0.00000000000000i\t-0.000354605101616778 + 0.998050063639308i\t0.00000000000000 + 0.00000000000000i\t-0.00156509993050963 - 1.00006401581498i\t0.00000000000000 + 0.00000000000000i\t-0.00379695600052438 - 1.00139885511569i\t0.00000000000000 + 0.00000000000000i\t0.000329023206098233 + 0.998352317884963i\t0.00000000000000 + 0.00000000000000i\t-0.000590902774422253 + 0.996840422969325i\t0.00000000000000 + 0.00000000000000i\t-0.00201336103373989 + 0.997462644900221i\t0.00000000000000 + 0.00000000000000i\t0.00118723852207253 + 0.997333792740890i\t0.00000000000000 + 0.00000000000000i\t-4.97899868873164e-06 - 0.997812309870580i\t0.00000000000000 + 0.00000000000000i\t0.00175276419797504 + 0.995284147275562i\t0.00000000000000 + 0.00000000000000i\t-0.00125204909784643 - 0.998480183830676i\t0.00000000000000 + 0.00000000000000i\t-0.000156161848597181 - 0.997875878331027i\t0.00000000000000 + 0.00000000000000i\t0.000915582181836960 + 0.997441223785563i\t0.00000000000000 + 0.00000000000000i\t-0.000714473378005121 + 0.999023750181081i\t0.00000000000000 + 0.00000000000000i\t0.000742692725197169 + 0.996640040451418i\t0.00000000000000 + 0.00000000000000i\t-0.000255762430226181 - 1.00071546328831i\t0.00000000000000 + 0.00000000000000i\t-0.00237644629731570 - 0.998103512910141i\t0.00000000000000 + 0.00000000000000i\t-0.00199897288585371 - 0.998207363125413i\t0.00000000000000 + 0.00000000000000i\t0.00106046474807930 - 0.997353689041293i\t0.00000000000000 + 0.00000000000000i\t-0.00196123730769182 - 1.00018118069824i\t0.00000000000000 + 0.00000000000000i\t0.00200702791234686 - 1.00022265537262i\t0.00000000000000 + 0.00000000000000i\t0.000303066330948121 + 1.00171302805839i\t0.00000000000000 + 0.00000000000000i\t-0.000858127766466321 - 0.996081051766369i\t0.00000000000000 + 0.00000000000000i\t-0.000574946392339404 - 0.996112866352626i])"  NumeratorPrototype=[]  FilterStructure=Direct form systolic  SerializationOption=Minimum number of cycles between valid input samples  NumCycles=2  NumberOfMultipliers=2  SimulateUsing=Code generation  roundingMode=Floor  overflowMode=off  CoefficientsDataTypeStr=Inherit: Same word length as input  OutputDataTypeStr=fixdt(1, 18, 13)  ResetInputPort=off  HDLGlobalReset=off
  Product : Product  OutDataTypeStr=Inherit: Same as first input
  Product1 : Product  OutDataTypeStr=Inherit: Same as first input
  SOF Correlation : dsphdlfiltering2/Discrete FIR Filter  NumeratorSource=Property  Numerator=flip([0.0000 - 1.0000i 0.0000 - 1.0000i 0.0000 - 1.0000i 0.0000 - 1.0000i 0.0000 + 1.0000i 0.0000 + 1.0000i 0.0000 + 1.0000i 0.0000 + 1.0000i 0.0000 - 1.0000i 0.0000 + 1.0000i 0.0000 + 1.0000i 0.0000 + 1.0000i 0.0000 - 1.0000i 0.0000 + 1.0000i 0.0000 + 1.0000i 0.0000 - 1.0000i 0.0000 - 1.0000i 0.0000 + 1.0000i 0.0000 - 1.0000i 0.0000 - 1.0000i 0.0000 + 1.0000i 0.0000 - 1.0000i 0.0000 + 1.0000i 0.0000 + 1.0000i 0.0000 - 1.0000i])  NumeratorPrototype=[]  FilterStructure=Direct form systolic  SerializationOption=Minimum number of cycles between valid input samples  NumCycles=2  NumberOfMultipliers=2  SimulateUsing=Code generation  roundingMode=Floor  overflowMode=off  CoefficientsDataTypeStr=Inherit: Same word length as input  OutputDataTypeStr=fixdt(1, 18, 13)  ResetInputPort=off  HDLGlobalReset=off
  Scope : Scope  NumInputPorts=2
  Scope1 : Scope  NumInputPorts=2
  Terminator : Terminator
  Terminator1 : Terminator
  SoFCorrelator : Outport
  PLSCCorrelator : Outport  Port=2
  Threshold : Outport  Port=3
  wires:
  Product/1 -> PLSC Correlation/1, SOF Correlation/1
  ValidIn/1 -> PLSC Correlation/2, SOF Correlation/2, MovingSum/3(ValidIn)
  DataIn/1 -> Math Function/1, Delay/1, Product1/1, Math Function1/1
  Math Function1/1 -> Product1/2
  PLSC Correlation/2 -> Terminator1/1
  Math Function/1 -> Product/1
  SOF Correlation/2 -> Terminator/1
  SOF Correlation/1 -> Delay1/1
  Product1/1 -> Complex to Real-Imag/1
  Delay/1 -> Product/2
  Complex to Real-Imag/1 -> Gain/1, Gain1/1
  MovingSum/1(E1) -> Scope1/1, Add/1
  MovingSum/2(E2) -> Scope1/2, Add/2
  Add/1 -> Threshold/1
  PLSC Correlation/1 -> PLSCCorrelator/1, Abs1/1
  Delay1/1 -> SoFCorrelator/1, Abs/1
  Gain/1 -> MovingSum/1(Scaled1)
  Gain1/1 -> MovingSum/2(Scaled2)
  Abs/1 -> Scope/1
  Abs1/1 -> Scope/2

== system PLFrameGenerator/FrameSynchronization/Correlator Sum and threshold scaling ==
  SOFCorr : Inport
  PLSCCorr : Inport  Port=2
  threshold : Inport  Port=3
  Complex to Real-Imag : ComplexToRealImag  Output=Real
  Complex to Real-Imag1 : ComplexToRealImag  Output=Real
  Conjugate : Math  Operator=conj  SignedPower=on  RndMeth=Zero
  Conjugate1 : Math  Operator=conj  SignedPower=on  RndMeth=Zero
  Corr Add : Sum
  Corr Subtract : Sum  Inputs=+-
  Delay : Delay  DelayLength=75
  Product : Product
  Product1 : Product
  Scope : Scope  NumInputPorts=3
  Sqrt : Sqrt  Commented=through
  Sqrt1 : Sqrt  Commented=through
  Threshold Scaling : Gain  Gain=0.6*debugHeaderGain^2  OutDataTypeStr=Inherit: Same as input
      mask init:
      | Simulink.suppressDiagnostic(gcb, 'SimulinkFixedPoint:util:fxpParameterPrecisionLoss');
  Correlation : Outport
  scaled_threshold : Outport  Port=2
  wires:
  PLSCCorr/1 -> Corr Add/2, Corr Subtract/2
  SOFCorr/1 -> Corr Subtract/1, Corr Add/1
  Corr Add/1 -> Product/1, Conjugate/1
  Conjugate/1 -> Product/2
  Product/1 -> Complex to Real-Imag/1
  Product1/1 -> Complex to Real-Imag1/1
  Conjugate1/1 -> Product1/2
  Corr Subtract/1 -> Product1/1, Conjugate1/1
  Complex to Real-Imag/1 -> Sqrt/1
  Complex to Real-Imag1/1 -> Sqrt1/1
  threshold/1 -> Threshold Scaling/1
  Sqrt/1 -> Correlation/1, Scope/1
  Sqrt1/1 -> Scope/2
  Threshold Scaling/1 -> Delay/1
  Delay/1 -> scaled_threshold/1

== system PLFrameGenerator/FrameSynchronization/Peak Detector ==
  Correlation : Inport
  scaled_threshold : Inport  Port=2
  Relational Operator : RelationalOperator  Operator=>  OutDataTypeStr=boolean  RndMeth=Simplest  InputSameDT=off
  thersholdExceeded : Outport
  wires:
  Correlation/1 -> Relational Operator/1
  Relational Operator/1 -> thersholdExceeded/1
  scaled_threshold/1 -> Relational Operator/2

== system PLFrameGenerator/FrameSynchronization/Peak Distance Detector ==
  note: Possible PLFrame lengths
      | 		   normal     short
      | QPSK        33282      8370
      | 16APSK    16686      4212
      |
      | DUMMY frame is always 3330
  Correlation : Inport
  16 APSK normal detector : Subsystem
  16 APSK short detector : Subsystem
  Decision Block : Subsystem
  Display{,1..8} (9 alike) : Display
  QPSK normal detector : Subsystem
  QPSK short detector : Subsystem
  EndOfSoF : Outport
  FrameSyncSuccess : Outport  Port=2
  PLFrameHDRValid : Outport  Port=3
  wires:
  Correlation/1 -> QPSK normal detector/1(Correlation), QPSK short detector/1(Correlation), 16 APSK short detector/1(Correlation), 16 APSK normal detector/1(Correlation)
  16 APSK short detector/1(Est. frame length) -> Display/1
  16 APSK normal detector/1(Est. window length) -> Display1/1
  QPSK short detector/1(Est. window length) -> Display2/1
  QPSK normal detector/1(Est. window length) -> Display3/1
  16 APSK short detector/2(Format Detected) -> Display4/1, Decision Block/1(16APSK short Valid)
  16 APSK normal detector/2(Format Detected) -> Decision Block/3(16APSK normal Valid), Display5/1
  QPSK short detector/2(Format Detected) -> Decision Block/5(QPSK short Valid), Display6/1
  QPSK normal detector/2(Format Detected) -> Decision Block/7(QPSK normal Valid), Display7/1
  16 APSK normal detector/3(StartOfSoF) -> Decision Block/4(16APSK normal start of SOF), Display8/1
  16 APSK short detector/3(StartOfSOF) -> Decision Block/2(16APSK short start of SOF)
  Decision Block/2(FrameSync success) -> FrameSyncSuccess/1
  Decision Block/1(EndOfSOD) -> EndOfSoF/1
  Decision Block/3(HeaderValid) -> PLFrameHDRValid/1
  QPSK short detector/3(StartOfSoF) -> Decision Block/6(QPSK short start of SOF)
  QPSK normal detector/3(StartOfSoF) -> Decision Block/8(QPSK normal start of SOF)

== system PLFrameGenerator/PL Descrambler and Pilot Valid Indicator/PL Data Descrambler ==
  note: The descrambler is currently with all ones (disabled)
      | To be implemented
  reset : Inport
  inputCount : Inport  Port=2
  validIn : Inport  Port=3
  dataIn : Inport  Port=4
  Compare To Constant1 : simulink/Logic and Bit Operations/Compare To Constant  relop=<=  const=PLSCLength-1  OutDataTypeStr=boolean
  Delay : Delay  DelayLength=54
  HDL Counter : hdlsllib/Sources/HDL Counter  CountType=Count limited  CountInit=0  CountStep=1  CountMax=25  CountFromType=Initial value  CountFrom=0  CountResetPort=on  CountLoadPort=off  CountEnbPort=on  CountDirPort=off  CountHitOutputPort=off  CountDataType=Unsigned  CountWordLen=8  CountFracLen=0  CountSampTime=1
  PL Scramble Sequence Mapper LUT : Lookup_n-D  NumberOfTableDimensions=1  LookupTableObject=''  BreakpointsSpecification=Even spacing  BreakpointsForDimension1=[-5:5]  BreakpointsForDimension1FirstPoint=0  BreakpointsForDimension2FirstPoint=10  BreakpointsForDimension2Spacing=12  IndexSearchMethod=Evenly spaced points  Table=ones(25, 1)  TableDataTypeStr=fixdt(1,2,0)  InterpMethod=Flat  DiagnosticForOutOfRangeInput=Error  InternalRulePriority=Speed  OutDataTypeStr=fixdt(1,2,0)  RndMeth=Simplest
  Product : Product  OutDataTypeStr=Inherit: Same as first input
  Switch : Switch  Criteria=u2 ~= 0  SaturateOnIntegerOverflow=off  InputSameDT=off
  dataOut : Outport
  valdiOut : Outport  Port=2
  wires:
  reset/1 -> HDL Counter/1
  inputCount/1 -> Compare To Constant1/1
  validIn/1 -> valdiOut/1, HDL Counter/2
  HDL Counter/1 -> PL Scramble Sequence Mapper LUT/1
  dataIn/1 -> Switch/1, Product/1
  PL Scramble Sequence Mapper LUT/1 -> Product/2
  Compare To Constant1/1 -> Switch/2
  Switch/1 -> Delay/1
  Product/1 -> Switch/3
  Delay/1 -> dataOut/1

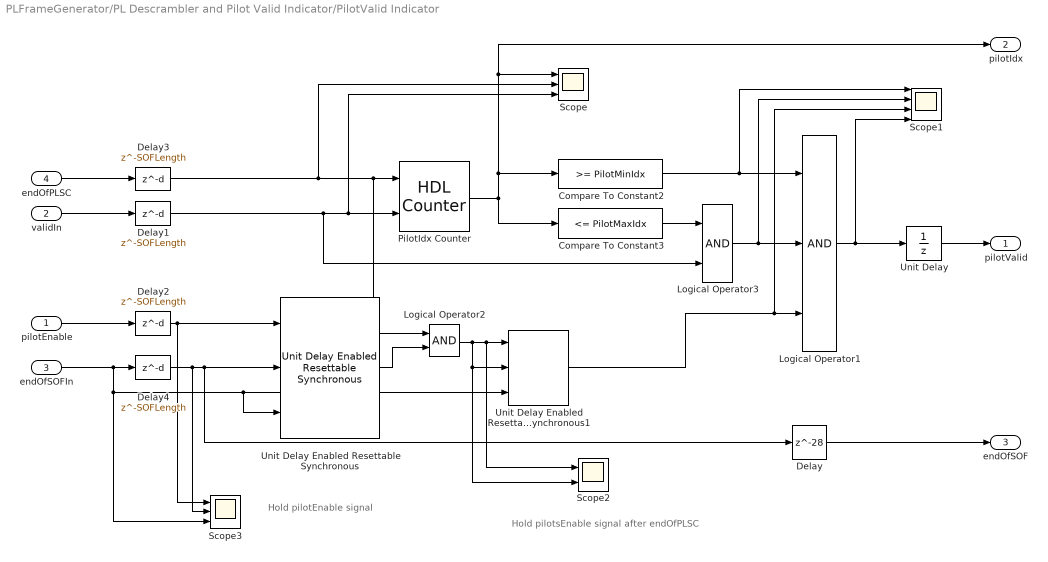
== system PLFrameGenerator/PL Descrambler and Pilot Valid Indicator/PilotValid Indicator ==
  note: Hold pilotEnable signal
  note: Hold pilotsEnable signal after endOfPLSC
  pilotEnable : Inport
  validIn : Inport  Port=2
  endOfSOFIn : Inport  Port=3
  endOfPLSC : Inport  Port=4
  Compare To Constant2 : simulink/Logic and Bit Operations/Compare To Constant  relop=>=  const=PilotMinIdx  OutDataTypeStr=boolean
  Compare To Constant3 : simulink/Logic and Bit Operations/Compare To Constant  relop=<=  const=PilotMaxIdx  OutDataTypeStr=boolean
  Delay : Delay  DelayLength=28
  Delay{1..4} (4 alike) : Delay  DelayLength=SOFLength
  Logical Operator1 : Logic  Inputs=3  AllPortsSameDT=off  OutDataTypeStr=boolean
  Logical Operator2 : Logic  AllPortsSameDT=off  OutDataTypeStr=boolean
  Logical Operator3 : Logic  AllPortsSameDT=off  OutDataTypeStr=boolean
  PilotIdx Counter : hdlsllib/Sources/HDL Counter  CountType=Count limited  CountInit=0  CountStep=1  CountMax=PilotMaxIdx  CountFromType=Initial value  CountFrom=0  CountResetPort=on  CountLoadPort=off  CountEnbPort=on  CountDirPort=off  CountHitOutputPort=off  CountDataType=Unsigned  CountWordLen=nextpow2(PilotMaxIdx)  CountFracLen=0  CountSampTime=1
  Scope : Scope  NumInputPorts=3
  Scope1 : Scope  NumInputPorts=4
  Scope2 : Scope  NumInputPorts=2
  Scope3 : Scope  NumInputPorts=3
  Unit Delay : UnitDelay  SampleTime=-1  HasFrameUpgradeWarning=on
  Unit Delay Enabled Resettable Synchronous : hdlsllib/Discrete/Unit Delay Enabled Resettable Synchronous  InitialCondition=0.0  SampleTime=1/Rsym
  Unit Delay Enabled Resettable Synchronous1 : hdlsllib/Discrete/Unit Delay Enabled Resettable Synchronous  InitialCondition=0.0  SampleTime=-1
  pilotValid : Outport
  pilotIdx : Outport  Port=2
  endOfSOF : Outport  Port=3
  wires:
  endOfPLSC/1 -> Delay3/1
  validIn/1 -> Delay1/1
  PilotIdx Counter/1 -> Scope/1, pilotIdx/1, Compare To Constant2/1, Compare To Constant3/1
  Compare To Constant2/1 -> Scope1/1, Logical Operator1/1
  Logical Operator1/1 -> Scope1/4, Unit Delay/1
  Compare To Constant3/1 -> Logical Operator3/1
  Logical Operator3/1 -> Scope1/2, Logical Operator1/2
  pilotEnable/1 -> Delay2/1
  Unit Delay Enabled Resettable Synchronous/1 -> Logical Operator2/2
  Logical Operator2/1 -> Scope2/2, Unit Delay Enabled Resettable Synchronous1/2, Scope2/1, Unit Delay Enabled Resettable Synchronous1/1
  Unit Delay Enabled Resettable Synchronous1/1 -> Scope1/3, Logical Operator1/3
  Delay3/1 -> Scope/2, Logical Operator2/1, PilotIdx Counter/1
  Delay1/1 -> Logical Operator3/2, Scope/3, PilotIdx Counter/2
  Delay2/1 -> Scope3/1, Unit Delay Enabled Resettable Synchronous/1
  endOfSOFIn/1 -> Scope3/3, Unit Delay Enabled Resettable Synchronous1/3, Unit Delay Enabled Resettable Synchronous/3, Delay4/1
  Delay4/1 -> Scope3/2, Delay/1, Unit Delay Enabled Resettable Synchronous/2
  Delay/1 -> endOfSOF/1
  Unit Delay/1 -> pilotValid/1

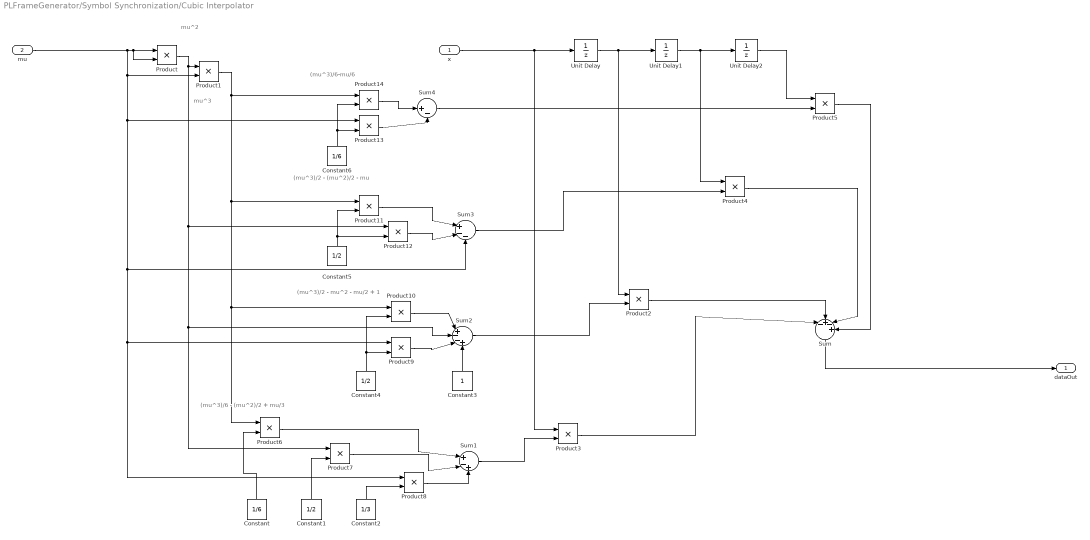
== system PLFrameGenerator/Symbol Synchronization/Cubic Interpolator ==
  note: (mu^3)/6-mu/6
  note: (mu^3)/2 - (mu^2)/2 - mu
  note: (mu^3)/2 - mu^2 - mu/2 + 1
  note: (mu^3)/6 - (mu^2)/2 + mu/3
  note: mu^2
  note: mu^3
  x : Inport
  mu : Inport  Port=2
  Constant : Constant  Value=1/6  SampleTime=-1
  Constant1 : Constant  Value=1/2  SampleTime=-1
  Constant2 : Constant  Value=1/3  SampleTime=-1
  Constant3 : Constant  SampleTime=-1
  Constant4 : Constant  Value=1/2  SampleTime=-1
  Constant5 : Constant  Value=1/2  SampleTime=-1
  Constant6 : Constant  Value=1/6  SampleTime=-1
  Product{,1..14} (15 alike) : Product
  Sum : Sum  Inputs=|-+-+
  Sum1 : Sum  Inputs=|+-+
  Sum2 : Sum  Inputs=|+--+
  Sum3 : Sum  Inputs=|+--
  Sum4 : Sum  Inputs=|+-
  Unit Delay : UnitDelay  SampleTime=-1  HasFrameUpgradeWarning=on
  Unit Delay1 : UnitDelay  SampleTime=-1  HasFrameUpgradeWarning=on
  Unit Delay2 : UnitDelay  SampleTime=-1  HasFrameUpgradeWarning=on
  dataOut : Outport
  wires:
  Sum/1 -> dataOut/1
  mu/1 -> Product/2, Product/1, Product13/1, Sum3/3, Product9/1, Product8/1, Product1/2
  Product/1 -> Product12/1, Sum2/2, Product7/1, Product1/1
  Unit Delay/1 -> Product2/1, Unit Delay1/1
  Unit Delay1/1 -> Product4/1, Unit Delay2/1
  Unit Delay2/1 -> Product5/1
  x/1 -> Product3/1, Unit Delay/1
  Product3/1 -> Sum/1
  Product2/1 -> Sum/2
  Product4/1 -> Sum/3
  Product5/1 -> Sum/4
  Constant/1 -> Product6/2
  Product1/1 -> Product11/1, Product10/1, Product6/1, Product14/1
  Constant1/1 -> Product7/2
  Constant2/1 -> Product8/2
  Product7/1 -> Sum1/2
  Sum1/1 -> Product3/2
  Product8/1 -> Sum1/3
  Product6/1 -> Sum1/1
  Constant3/1 -> Sum2/4
  Constant4/1 -> Product10/2, Product9/2
  Product9/1 -> Sum2/3
  Product10/1 -> Sum2/1
  Sum2/1 -> Product2/2
  Constant5/1 -> Product11/2, Product12/2
  Product12/1 -> Sum3/2
  Product11/1 -> Sum3/1
  Sum3/1 -> Product4/2
  Constant6/1 -> Product14/2, Product13/2
  Product14/1 -> Sum4/1
  Product13/1 -> Sum4/2
  Sum4/1 -> Product5/2

== system PLFrameGenerator/Symbol Synchronization/Linear Interpolator ==
  x : Inport
  mu : Inport  Port=2
  Buffer : Buffer  N=2  OutputFrames=off
  Constant : Constant  SampleTime=-1
  Product : Product
  Sum : Sum  Inputs=|+-
  Sum1 : Sum  Inputs=|++
  Sum2 : Sum  Inputs=|++
  Unbuffer : Unbuffer
  Unit Delay : UnitDelay  SampleTime=-1  HasFrameUpgradeWarning=on
  dataOut : Outport
  wires:
  Unit Delay/1 -> Sum/2, Sum2/1
  Sum1/1 -> Product/2
  Sum/1 -> Product/1
  mu/1 -> Sum1/1
  Sum2/1 -> Unbuffer/1
  x/1 -> Buffer/1
  Constant/1 -> Sum1/2
  Product/1 -> Sum2/2
  Buffer/1 -> Sum/1, Unit Delay/1
  Unbuffer/1 -> dataOut/1

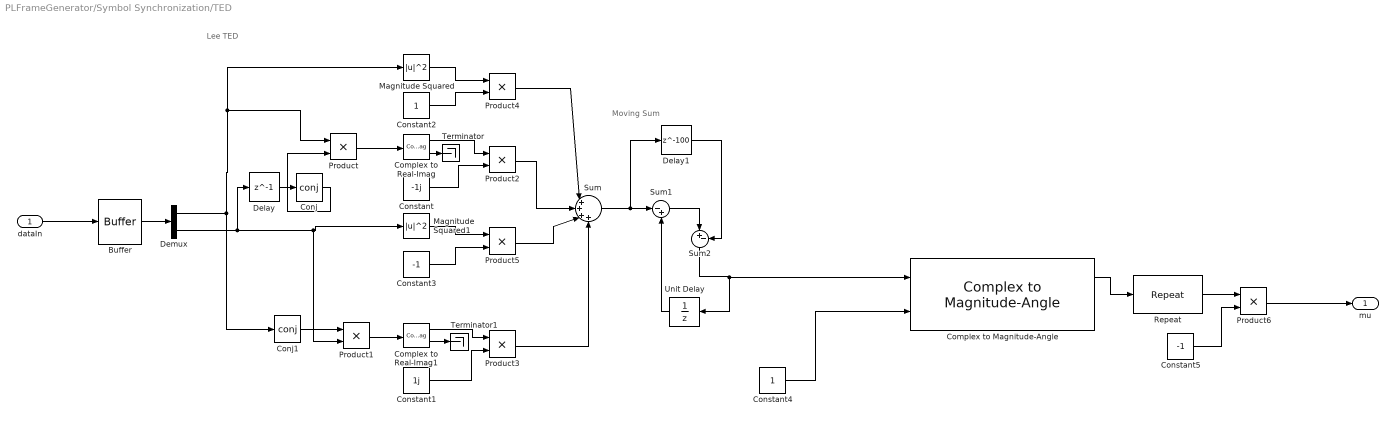
== system PLFrameGenerator/Symbol Synchronization/TED ==
  note: Lee TED
  note: Moving Sum
  dataIn : Inport
  Buffer : Buffer  N=2  OutputFrames=off
  Complex to Real-Imag : ComplexToRealImag
  Complex to Real-Imag1 : ComplexToRealImag
  Complex to Magnitude-Angle : dsphdlmathfun2/Complex to Magnitude-Angle  NumIterationsSource=Auto  NumIterations=10  OutputFormat=Angle  AngleFormat=Normalized  ScaleOutput=on  ScalingMethod=Shift-Add  SimulateUsing=Code generation
  Conj : Math  Operator=conj
  Conj1 : Math  Operator=conj
  Constant : Constant  Value=-1j  SampleTime=1/Rsym
  Constant1 : Constant  Value=1j  SampleTime=1/Rsym
  Constant2 : Constant  SampleTime=1/Rsym
  Constant3 : Constant  Value=-1  SampleTime=1/Rsym
  Constant4 : Constant  OutDataTypeStr=boolean  SampleTime=1/Rsym
  Constant5 : Constant  Value=-1  SampleTime=1/2/Rsym
  Delay : Delay  DelayLength=1  InitialCondition=0
  Delay1 : Delay  DelayLength=100
  Demux : Demux  Outputs=2
  Magnitude Squared : Math  Operator=magnitude^2
  Magnitude Squared1 : Math  Operator=magnitude^2
  Product{,1..5} (6 alike) : Product
  Product6 : Product  OutDataTypeStr=double
  Repeat : dspsigops/Repeat  FactorSource=Dialog parameter  N=2  Nmax=16  InputProcessing=Columns as channels (frame based)  RateOptions=Allow multirate processing  ic=0  mode=Unused parameter value
      settings: LibrarySourceBlock=commsequence2/Repeat
  Sum : Sum  Inputs=|++++
  Sum1 : Sum  Inputs=|-+
  Sum2 : Sum  Inputs=|+-
  Terminator : Terminator
  Terminator1 : Terminator
  Unit Delay : UnitDelay  SampleTime=-1  HasFrameUpgradeWarning=on
  mu : Outport
  wires:
  Product4/1 -> Sum/1
  Complex to Real-Imag1/2 -> Terminator1/1
  Sum1/1 -> Sum2/1
  Constant1/1 -> Product3/2
  Product3/1 -> Sum/4
  Conj/1 -> Product/2
  Complex to Real-Imag/2 -> Terminator/1
  Conj1/1 -> Product1/1
  Delay1/1 -> Sum2/2
  Delay/1 -> Conj/1
  Sum2/1 -> Unit Delay/1, Complex to Magnitude-Angle/1
  Constant3/1 -> Product5/2
  Sum/1 -> Sum1/1, Delay1/1
  Complex to Real-Imag1/1 -> Product3/1
  Product/1 -> Complex to Real-Imag/1
  Product1/1 -> Complex to Real-Imag1/1
  Complex to Real-Imag/1 -> Product2/1
  Magnitude Squared1/1 -> Product5/1
  Constant/1 -> Product2/2
  Unit Delay/1 -> Sum1/2
  Constant2/1 -> Product4/2
  Product2/1 -> Sum/2
  Product5/1 -> Sum/3
  dataIn/1 -> Buffer/1
  Magnitude Squared/1 -> Product4/1
  Demux/1 -> Product/1, Magnitude Squared/1, Conj1/1
  Constant4/1 -> Complex to Magnitude-Angle/2
  Buffer/1 -> Demux/1
  Demux/2 -> Delay/1, Product1/2, Magnitude Squared1/1
  Repeat/1 -> Product6/1
  Product6/1 -> mu/1
  Constant5/1 -> Product6/2
  Complex to Magnitude-Angle/1 -> Repeat/1

== system PLFrameGenerator/Symbol Synchronization/unwrapper ==
  In1 : Inport
  Output : Outport
  wires:
  In1/1 -> Output/1

== system PLFrameGenerator/FrameSynchronization/Correlator/MovingSum ==
  note: Delay by length of SoF sequence
  Scaled1 : Inport
  Scaled2 : Inport  Port=2
  ValidIn : Inport  Port=3
  Add : Sum  Inputs=|+-  OutDataTypeStr=Inherit: Same as first input
  Add1 : Sum  Inputs=|++  OutDataTypeStr=Inherit: Same as first input
  Add2 : Sum  Inputs=|+-  OutDataTypeStr=Inherit: Same as first input
  Add3 : Sum  Inputs=|++  OutDataTypeStr=Inherit: Same as first input
  Delay : Delay  DelayLength=26  ShowEnablePort=on
      settings: InputPortMap=u0,e6
  Delay1 : Delay  DelayLength=64  ShowEnablePort=on
      settings: InputPortMap=u0,e6
  Delay14 : Delay  DelayLength=1  ShowEnablePort=on
      settings: InputPortMap=u0,e6
  Delay2 : Delay  DelayLength=1  ShowEnablePort=on
      settings: InputPortMap=u0,e6
  E1 : Outport
  E2 : Outport  Port=2
  wires:
  Scaled1/1 -> Add/1, Delay/1
  Delay/1 -> Add/2
  Add/1 -> Add1/1
  Delay14/1 -> Add1/2
  Scaled2/1 -> Delay1/1, Add2/1
  Delay1/1 -> Add2/2
  ValidIn/1 -> Delay1/2, Delay/2, Delay14/2, Delay2/2
  Add2/1 -> Add3/1
  Delay2/1 -> Add3/2
  Add3/1 -> Delay2/1, E2/1
  Add1/1 -> E1/1, Delay14/1
